simulink model "aoo"  (R2020a)
settings: Solver=FixedStepAuto  StartTime=0.0  StopTime=10.0  FixedStep=1e-3  RelTol=1e-3  EnableMultiTasking=on
undefined symbols (not defined in the file): D10, D11, D12, D2, D4, D5, D7, D8, D9, PTA0, PTA2, PTB23, PTB9, PTC3, PTC4, PTD0, PTD2, PTD3
libraries: frdmk64flib x10
settings Model: ExtModeTrigDuration=5  Creator=raymo  LastModifiedBy=raymo
settings OptimizationCC: EnhancedBackFolding=on  PassReuseOutputArgsAs=Individual arguments  ZeroExternalMemoryAtStartup=off  ZeroInternalMemoryAtStartup=off  MaxStackSize=64  OptimizeBlockOrder=speed  DifferentSizesBufferReuse=on  OptimizationCustomize=off  EfficientTunableParamExpr=on
settings DebuggingCC: ParameterTunabilityLossMsg=error
settings HardwareCC: ProdBitPerPointer=32  ProdBitPerSizeT=32  ProdBitPerPtrDiffT=32  ProdLargestAtomicInteger=Long  ProdLargestAtomicFloat=Double  ProdWordSize=32  ProdHWDeviceType=ARM Compatible->ARM Cortex
settings SFSimCC: MATLABDynamicMemAlloc=off
settings RTWCC: SystemTargetFile=ert.tlc  HardwareBoard=NXP FRDM-K64F  TemplateMakefile=ert_default_tmf  Toolchain=GNU Tools for ARM Embedded Processors
settings CodeAppCC: ForceParamTrailComments=on  IgnoreCustomStorageClasses=off  OperatorAnnotations=on  SimulinkDataObjDesc=on  SFDataObjDesc=on  InsertBlockDesc=on

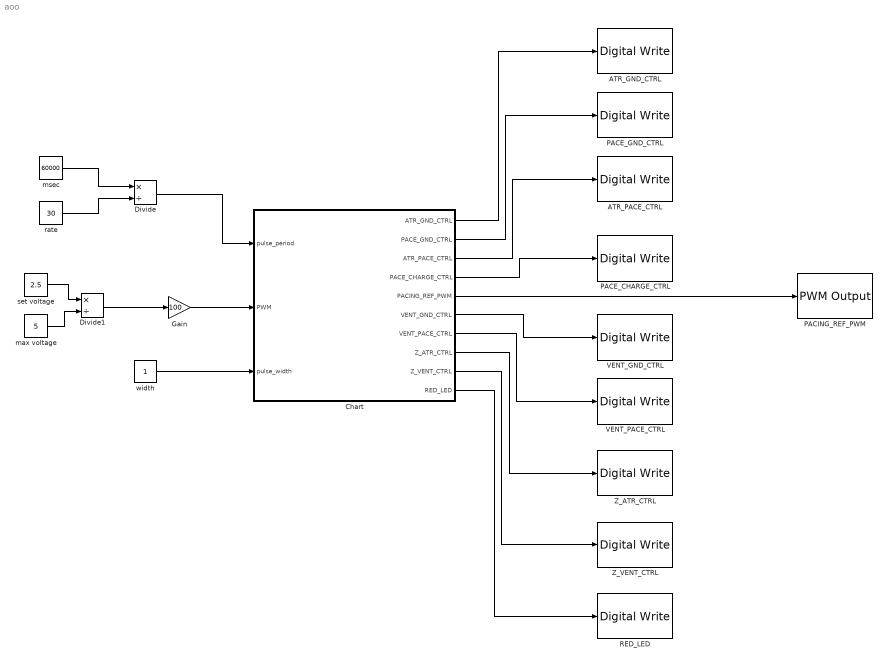
== system aoo ==
  ATR_GND_CTRL : frdmk64flib/Digital Write  Whichpin=PTD2 (D11)
  ATR_PACE_CTRL : frdmk64flib/Digital Write  Whichpin=PTA0 (D8)
  Chart : Stateflow chart  TreatAsAtomicUnit=on
  Divide : Product  Inputs=*/
  Divide1 : Product  Inputs=*/
  Gain : Gain  Gain=100
  PACE_CHARGE_CTRL : frdmk64flib/Digital Write  Whichpin=PTB9 (D2)
  PACE_GND_CTRL : frdmk64flib/Digital Write  Whichpin=PTD0 (D10)
  PACING_REF_PWM : frdmk64flib/PWM Output  Whichpin=PTA2 (D5)  InitialFrequency=2000  InitialDutyCycle=50
  RED_LED : frdmk64flib/Digital Write  Whichpin=RED_LED
  VENT_GND_CTRL : frdmk64flib/Digital Write  Whichpin=PTD3 (D12)
  VENT_PACE_CTRL : frdmk64flib/Digital Write  Whichpin=PTC4 (D9)
  Z_ATR_CTRL : frdmk64flib/Digital Write  Whichpin=PTB23 (D4)
  Z_VENT_CTRL : frdmk64flib/Digital Write  Whichpin=PTC3 (D7)
  max voltage : Constant  Value=5
  msec : Constant  Value=60000
  rate : Constant  Value=30
  set voltage : Constant  Value=2.5
  width : Constant
  wires:
  Divide/1 -> Chart/1(pulse_period)
  Chart/5(PACING_REF_PWM) -> PACING_REF_PWM/1
  Chart/1(ATR_GND_CTRL) -> ATR_GND_CTRL/1
  Chart/2(PACE_GND_CTRL) -> PACE_GND_CTRL/1
  Chart/3(ATR_PACE_CTRL) -> ATR_PACE_CTRL/1
  Chart/4(PACE_CHARGE_CTRL) -> PACE_CHARGE_CTRL/1
  Chart/6(VENT_GND_CTRL) -> VENT_GND_CTRL/1
  Chart/7(VENT_PACE_CTRL) -> VENT_PACE_CTRL/1
  Chart/8(Z_ATR_CTRL) -> Z_ATR_CTRL/1
  Chart/9(Z_VENT_CTRL) -> Z_VENT_CTRL/1
  msec/1 -> Divide/1
  rate/1 -> Divide/2
  width/1 -> Chart/3(pulse_width)
  Chart/10(RED_LED) -> RED_LED/1
  set voltage/1 -> Divide1/1
  max voltage/1 -> Divide1/2
  Divide1/1 -> Gain/1
  Gain/1 -> Chart/2(PWM)

== stateflow chart aoo/Chart ==
  state ChargeDishcharge
    entry:
    %C22
    ATR_PACE_CTRL = false;
    VENT_PACE_CTRL = false;
    PACING_REF_PWM = PWM;
    PACE_CHARGE_CTRL = true;
    %C21
    PACE_GND_CTRL = true;
    VENT_PACE_CTRL = false;
    Z_ATR_CTRL = false;
    Z_VENT_CTRL = false;
    ATR_GND_CTRL = true;
    VENT_GND_CTRL = false;
    %RED LED
    RED_LED = false;
  state AVpacing
    entry:
    PACE_CHARGE_CTRL = false;
    PACE_GND_CTRL = true;
    ATR_PACE_CTRL = true;
    ATR_GND_CTRL = false;
    Z_ATR_CTRL = false;
    Z_VENT_CTRL = false;
    VENT_GND_CTRL = false;
    VENT_PACE_CTRL = false;
    PACING_REF_PWM = PWM;
    RED_LED = true;
  (default) -> ChargeDishcharge
  AVpacing -> ChargeDishcharge : [after(pulse_width, msec)]
  ChargeDishcharge -> AVpacing : [after(pulse_period-pulse_width, msec)]
  data: ATR_GND_CTRL output; PACE_GND_CTRL output; ATR_PACE_CTRL output; PACE_CHARGE_CTRL output; PACING_REF_PWM output; VENT_GND_CTRL output; VENT_PACE_CTRL output; Z_ATR_CTRL output; Z_VENT_CTRL output; pulse_period input; PWM input; pulse_width input; RED_LED output
